simulink model "step"  (R2018b)
settings: Solver=VariableStepAuto  StartTime=0.0  StopTime=10.0  RelTol=1e-3
settings Model: Creator=frodan  LastModifiedBy=frodan

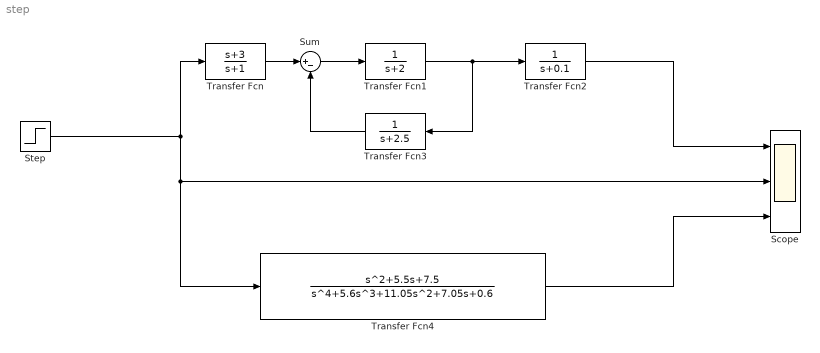
== system step ==
  Scope : Scope  NumInputPorts=3
  Step : Step  SampleTime=0
  Sum : Sum  Inputs=|+-
  Transfer Fcn : TransferFcn  Numerator=[1 3]  Denominator=[1 1]
  Transfer Fcn1 : TransferFcn  Denominator=[1 2]
  Transfer Fcn2 : TransferFcn  Denominator=[1 0.1]
  Transfer Fcn3 : TransferFcn  Denominator=[1 2.5]
  Transfer Fcn4 : TransferFcn  Numerator=[1 5.5 7.5]  Denominator=[1 5.6 11.05 7.05 0.6]
  wires:
  Step/1 -> Scope/2, Transfer Fcn4/1, Transfer Fcn/1
  Transfer Fcn1/1 -> Transfer Fcn3/1, Transfer Fcn2/1
  Transfer Fcn3/1 -> Sum/2
  Transfer Fcn/1 -> Sum/1
  Sum/1 -> Transfer Fcn1/1
  Transfer Fcn2/1 -> Scope/1
  Transfer Fcn4/1 -> Scope/3
